simulink model "openloop_sim"  (R2024a)
settings: Solver=VariableStepAuto  StartTime=0.0  StopTime=10.0  RelTol=1e-3
undefined symbols (not defined in the file): U0, X0
settings Model: Creator=mkaarthi  LastModifiedBy=mkaarthi

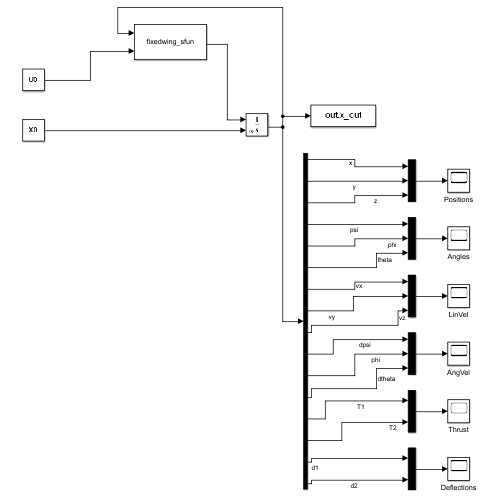
[thumbnail: Simulink's stored preview of the top-level diagram]
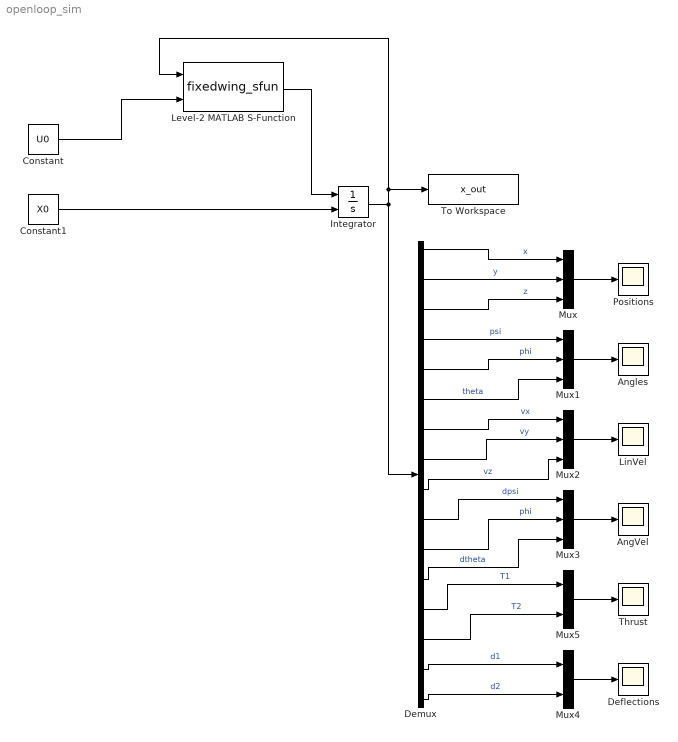
== system openloop_sim ==
  AngVel : Scope
  Angles : Scope
  Constant : Constant  Value=U0
  Constant1 : Constant  Value=X0
  Deflections : Scope
  Demux : Demux  Outputs=16
  Integrator : Integrator  InitialConditionSource=external
  Level-2 MATLAB S-Function : M-S-Function  FunctionName=fixedwing_sfun
  LinVel : Scope
  Mux{,1..3} (4 alike) : Mux  Inputs=3
  Mux4 : Mux  Inputs=2
  Mux5 : Mux  Inputs=2
  Positions : Scope
  Thrust : Scope
  To Workspace : ToWorkspace  VariableName=x_out  SampleTime=-1
  wires:
  Level-2 MATLAB S-Function/1 -> Integrator/1
  Constant/1 -> Level-2 MATLAB S-Function/2
  Integrator/1 -> Demux/1, To Workspace/1, Level-2 MATLAB S-Function/1
  Constant1/1 -> Integrator/2
  Demux/1 -> Mux/1  "x"
  Demux/2 -> Mux/2  "y"
  Demux/3 -> Mux/3  "z"
  Demux/5 -> Mux1/2  "phi"
  Demux/4 -> Mux1/1  "psi"
  Demux/6 -> Mux1/3  "theta"
  Demux/7 -> Mux2/1  "vx"
  Demux/8 -> Mux2/2  "vy"
  Demux/9 -> Mux2/3  "vz"
  Demux/12 -> Mux3/3  "dtheta"
  Demux/10 -> Mux3/1  "dpsi"
  Demux/11 -> Mux3/2  "phi"
  Demux/16 -> Mux4/2  "d2"
  Demux/15 -> Mux4/1  "d1"
  Demux/13 -> Mux5/1  "T1"
  Demux/14 -> Mux5/2  "T2"
  Mux/1 -> Positions/1
  Mux1/1 -> Angles/1
  Mux2/1 -> LinVel/1
  Mux3/1 -> AngVel/1
  Mux5/1 -> Thrust/1
  Mux4/1 -> Deflections/1
